simulink model "ysw11_7"  (R2014a)
settings: Solver=ode45  StartTime=0.0  StopTime=10.0  RelTol=1e-3
libraries: commanapbnd3 x1
settings Model: Creator=ii  LastModifiedBy=ii
settings SolverCC: ZeroCrossAlgorithm=Adaptive
settings DebuggingCC: UnderspecifiedInitializationDetection=Classic

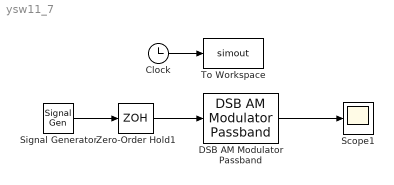
== system ysw11_7 ==
  Clock : Clock
  DSB AM Modulator Passband : commanapbnd3/DSB AM Modulator Passband  Fc=300  Ph=pi/3  Offset=100
  Scope1 : Scope
  Signal Generator : SignalGenerator  Frequency=700  Units=rad/sec
  To Workspace : ToWorkspace  VariableName=simout  SampleTime=-1
  Zero-Order Hold1 : ZeroOrderHold
  wires:
  Clock/1 -> To Workspace/1
  Signal Generator/1 -> Zero-Order Hold1/1
  Zero-Order Hold1/1 -> DSB AM Modulator Passband/1
  DSB AM Modulator Passband/1 -> Scope1/1
